simulink model "ecg_filter"  (R2026a)
settings: Solver=VariableStepAuto  StopTime=T_sim
values from neighbouring files (symbols this model uses):
  amp_heart = 1.0    (= 1)    [init_parameters.m]
  amp_noise = 0.4    [init_parameters.m]
  f_heart = 1.5    [init_parameters.m]
  f_noise = 50    [init_parameters.m]
undefined symbols (not defined in the file or in its folder): den_coeff, num_coeff
settings Model: Creator=khalo  LastModifiedBy=khalo

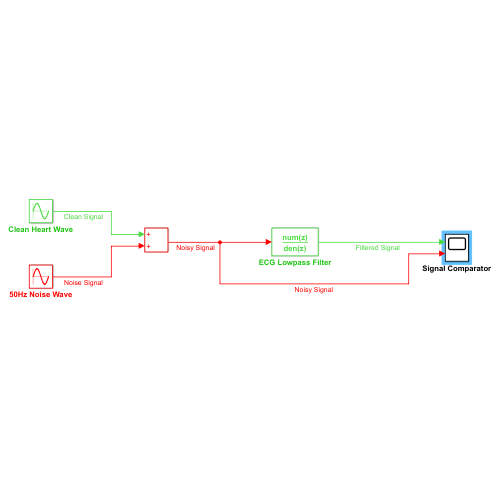
[thumbnail: Simulink's stored preview of the top-level diagram]
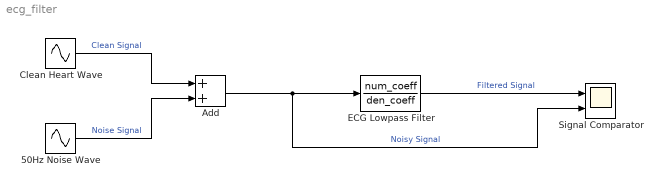
== system ecg_filter ==
  50Hz Noise Wave : Sin  Amplitude=amp_noise  Frequency=2*pi*f_noise  SampleTime=0
  Add : Sum
  Clean Heart Wave : Sin  Amplitude=amp_heart  Frequency=2*pi*f_heart  SampleTime=0
  ECG Lowpass Filter : DiscreteFilter  Numerator=num_coeff  Denominator=den_coeff
  Signal Comparator : Scope  NumInputPorts=2
      settings: ActiveDisplayYMinimum=-1.6830127018922179  ActiveDisplayYMaximum=1.6830127018922185
  wires:
  Clean Heart Wave/1 -> Add/1  "Clean Signal"
  50Hz Noise Wave/1 -> Add/2  "Noise Signal"
  Add/1 -> Signal Comparator/2, ECG Lowpass Filter/1  "Noisy Signal"
  ECG Lowpass Filter/1 -> Signal Comparator/1  "Filtered Signal"
